simulink model "dlb_sm"  (R2023a)
settings: Solver=FixedStepAuto  StartTime=0.0  StopTime=10.0  FixedStep=1e-6  RelTol=1e-3
settings Model: Creator=Zenos  LastModifiedBy=Zenos

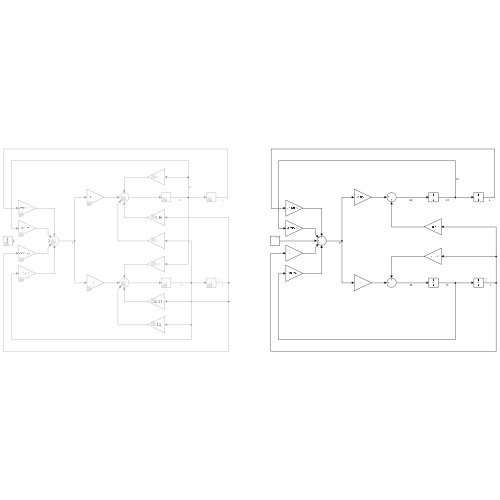
[thumbnail: Simulink's stored preview of the top-level diagram]
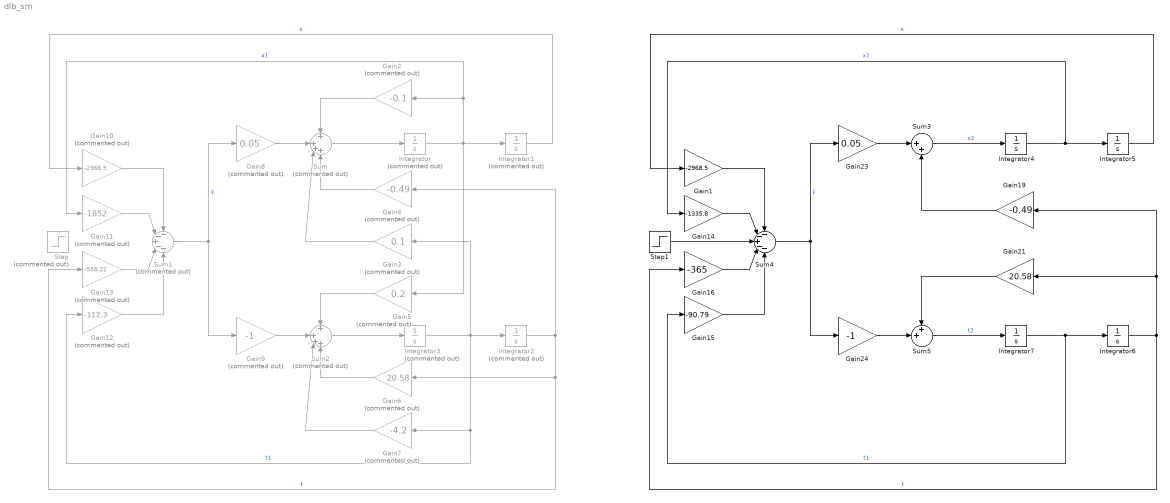
== system dlb_sm ==
  Gain1 : Gain  Gain=-2968.5
  Gain10 : Gain  Commented=on  Gain=-2968.5
  Gain11 : Gain  Commented=on  Gain=-1852
  Gain12 : Gain  Commented=on  Gain=-112.3
  Gain13 : Gain  Commented=on  Gain=-558.22
  Gain14 : Gain  Gain=-1335.8
  Gain15 : Gain  Gain=-90.79
  Gain16 : Gain  Gain=-365
  Gain19 : Gain  Gain=-0.49
  Gain2 : Gain  Commented=on  Gain=-0.1
  Gain21 : Gain  Gain=20.58
  Gain23 : Gain  Gain=0.05
  Gain24 : Gain  Gain=-1
  Gain3 : Gain  Commented=on  Gain=0.1
  Gain4 : Gain  Commented=on  Gain=-0.49
  Gain5 : Gain  Commented=on  Gain=0.2
  Gain6 : Gain  Commented=on  Gain=20.58
  Gain7 : Gain  Commented=on  Gain=-4.2
  Gain8 : Gain  Commented=on  Gain=0.05
  Gain9 : Gain  Commented=on  Gain=-1
  Integrator : Integrator  Commented=on
  Integrator1 : Integrator  Commented=on
  Integrator2 : Integrator  Commented=on  InitialCondition=0.1
  Integrator3 : Integrator  Commented=on
  Integrator4 : Integrator
  Integrator5 : Integrator
  Integrator6 : Integrator  InitialCondition=0.1
  Integrator7 : Integrator
  Step : Step  Commented=on  Time=4  After=100  SampleTime=0
  Step1 : Step  Time=4  After=100  SampleTime=0
  Sum : Sum  Commented=on  Inputs=+|+++
  Sum1 : Sum  Commented=on  Inputs=--+--
  Sum2 : Sum  Commented=on  Inputs=+|+++
  Sum3 : Sum  Inputs=|++
  Sum4 : Sum  Inputs=--+--
  Sum5 : Sum  Inputs=++|
  wires:
  Integrator/1 -> Gain11/1, Gain2/1, Gain5/1, Integrator1/1  "x1"
  Integrator3/1 -> Gain12/1, Gain7/1, Integrator2/1, Gain3/1  "t1"
  Integrator2/1 -> Gain13/1, Gain6/1, Gain4/1  "t"
  Sum/1 -> Integrator/1
  Gain2/1 -> Sum/1
  Gain3/1 -> Sum/3
  Gain4/1 -> Sum/4
  Gain5/1 -> Sum2/1
  Sum2/1 -> Integrator3/1
  Gain6/1 -> Sum2/4
  Gain7/1 -> Sum2/3
  Gain8/1 -> Sum/2
  Gain9/1 -> Sum2/2
  Sum1/1 -> Gain9/1, Gain8/1  "F"
  Integrator1/1 -> Gain10/1  "x"
  Gain10/1 -> Sum1/1
  Gain11/1 -> Sum1/2
  Gain13/1 -> Sum1/4
  Gain12/1 -> Sum1/5
  Gain1/1 -> Sum4/1
  Gain14/1 -> Sum4/2
  Gain15/1 -> Sum4/5
  Integrator7/1 -> Integrator6/1, Gain15/1  "t1"
  Integrator5/1 -> Gain1/1  "x"
  Sum3/1 -> Integrator4/1  "x2"
  Gain23/1 -> Sum3/1
  Sum4/1 -> Gain24/1, Gain23/1  "F"
  Gain24/1 -> Sum5/2
  Sum5/1 -> Integrator7/1  "t2"
  Integrator6/1 -> Gain21/1, Gain19/1, Gain16/1  "t"
  Gain16/1 -> Sum4/4
  Integrator4/1 -> Gain14/1, Integrator5/1  "x1"
  Gain21/1 -> Sum5/1
  Gain19/1 -> Sum3/2
  Step1/1 -> Sum4/3
